simulink model "mainModel"  (R2017a)
settings: Solver=VariableStepAuto  StartTime=0.0  StopTime=10.0  RelTol=1e-3
settings Model: Creator=manoj  LastModifiedBy=manoj

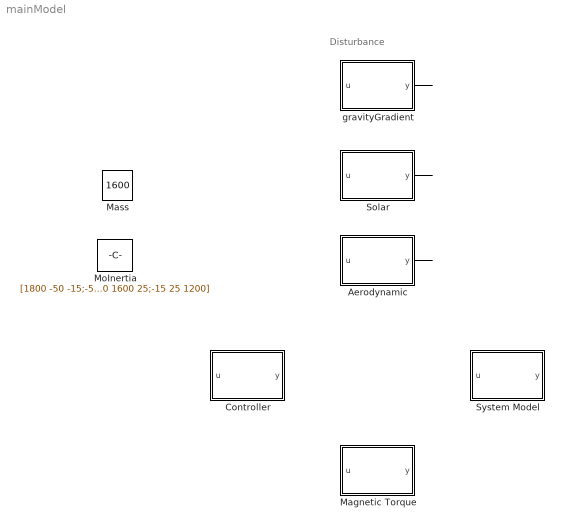
== system mainModel ==
  note: Disturbance
  "Aerodynamic " : MATLAB Function  TreatAsAtomicUnit=on
  "Controller " : MATLAB Function  TreatAsAtomicUnit=on
  "Magnetic Torque " : MATLAB Function  TreatAsAtomicUnit=on
  Mass : Constant  Value=1600
  "MoInertia " : Constant  Value=[1800 -50 -15;-50 1600 25;-15 25 1200]
  "Solar " : MATLAB Function  TreatAsAtomicUnit=on
  System Model : MATLAB Function  TreatAsAtomicUnit=on
  "gravityGradient " : MATLAB Function  TreatAsAtomicUnit=on
  wires:
  ? -> "Aerodynamic "/1(u)
  "Solar "/1(y) -> ?
  ? -> "Solar "/1(u)
  "gravityGradient "/1(y) -> ?
  ? -> "gravityGradient "/1(u)
  "Aerodynamic "/1(y) -> ?

== matlab function mainModel/Controller  ==
  data: u input; y output
function y = fcn(u)

y = u;

== matlab function mainModel/System Model ==
  data: u input; y output
function y = fcn(u)

y = u;

== matlab function mainModel/gravityGradient  ==
  data: u input; y output
function y = fcn(u)

y = u;

== matlab function mainModel/Solar  ==
  data: u input; y output
function y = fcn(u)

y = u;

== matlab function mainModel/Aerodynamic  ==
  data: u input; y output
function y = fcn(u)

y = u;

== matlab function mainModel/Magnetic Torque  ==
  data: u input; y output
function y = fcn(u)

y = u;
